simulink model "Enum"  (R2021a)
settings: Solver=VariableStepAuto  StartTime=0.0  StopTime=10.0  RelTol=1e-3
settings Model: Creator=omar  LastModifiedBy=omar

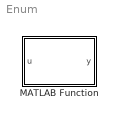
== system Enum ==
  MATLAB Function : MATLAB Function  TreatAsAtomicUnit=on

== matlab function Enum/MATLAB Function ==
  data: u input; y output
function y = fcn(u)
classdef LEDcolor < Simulink.IntEnumType
    enumeration
        RED
        GREEN
        BLUE
    end
end
